simulink model "ver8_1"  (R2020b)
settings: Solver=VariableStepAuto  StartTime=0.0  StopTime=10.0  RelTol=1e-3
undefined symbols (not defined in the file): c1, c3, c4, fn, j, m, r, v0, w0
settings Model: Creator=K E S SRINIVAS  LastModifiedBy=K E S SRINIVAS

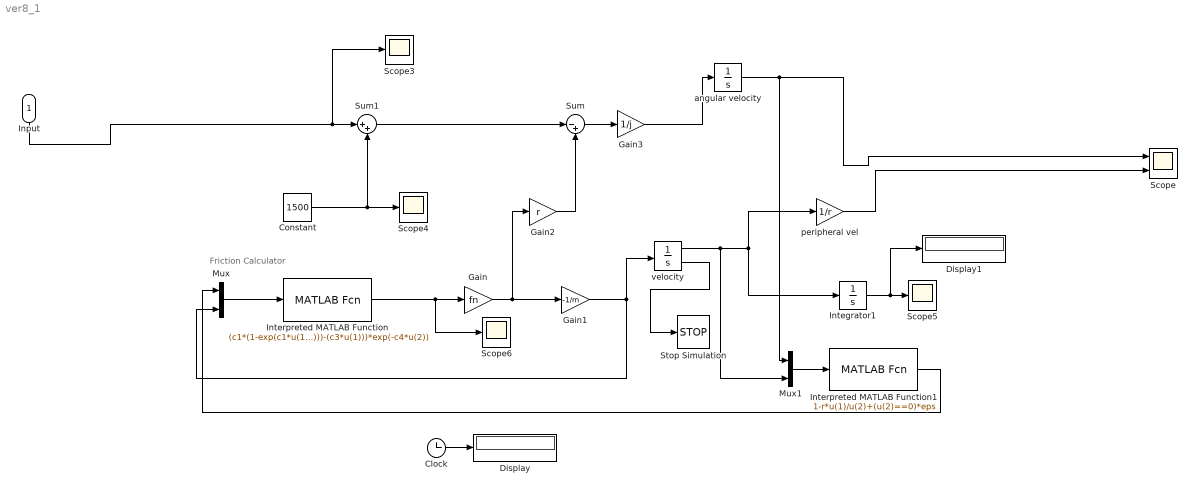
== system ver8_1 ==
  note: Friction Calculator
  Input : Inport
  Clock : Clock
  Constant : Constant  Value=1500
  Display : Display
  Display1 : Display
  Gain : Gain  Gain=fn
  Gain1 : Gain  Gain=-1/m
  Gain2 : Gain  Gain=r
  Gain3 : Gain  Gain=1/j
  Integrator1 : Integrator
  Interpreted MATLAB Function : MATLABFcn  MATLABFcn=(c1*(1-exp(c1*u(1)))-(c3*u(1)))*exp(-c4*u(2))  OutputDimensions=1
  Interpreted MATLAB Function1 : MATLABFcn  MATLABFcn=1-r*u(1)/u(2)+(u(2)==0)*eps  OutputDimensions=1
  Mux : Mux  Inputs=2
  Mux1 : Mux  Inputs=2
  Scope : Scope  NumInputPorts=2
  Scope{3..6} (4 alike) : Scope
  Stop Simulation : Stop
  Sum : Sum  Inputs=|-+
  Sum1 : Sum  Inputs=|++
  angular velocity : Integrator  InitialCondition=w0  LimitOutput=on  UpperSaturationLimit=1000  LowerSaturationLimit=0
  peripheral vel : Gain  Gain=1/r
  velocity : Integrator  InitialCondition=v0  LimitOutput=on  UpperSaturationLimit=1000  LowerSaturationLimit=0  ShowSaturationPort=on
  wires:
  Gain1/1 -> Mux/2, velocity/1
  Interpreted MATLAB Function/1 -> Scope6/1, Gain/1
  Mux/1 -> Interpreted MATLAB Function/1
  Gain/1 -> Gain2/1, Gain1/1
  velocity/1 -> Mux1/2, Integrator1/1, peripheral vel/1
  Gain2/1 -> Sum/2
  Sum/1 -> Gain3/1
  Gain3/1 -> angular velocity/1
  angular velocity/1 -> Mux1/1, Scope/1
  velocity/2 -> Stop Simulation/1
  peripheral vel/1 -> Scope/2
  Constant/1 -> Scope4/1, Sum1/2
  Sum1/1 -> Sum/1
  Input/1 -> Scope3/1, Sum1/1
  Integrator1/1 -> Display1/1, Scope5/1
  Clock/1 -> Display/1
  Interpreted MATLAB Function1/1 -> Mux/1
  Mux1/1 -> Interpreted MATLAB Function1/1
